simulink model "model_in_simulink"  (R2017a)
settings: Solver=FixedStepAuto  StartTime=0.0  StopTime=36*5  FixedStep=0.005  RelTol=1e-3
values from neighbouring files (symbols this model uses):
  a = theta(:,6)    [estimate_BP.m]
  alpha_Gain = theta(:,1)    [estimate_BP.m]
  alpha_Loss = theta(:,2)    [estimate_BP.m]
  b = theta(:,7)    [estimate_BP.m]
  beta_v = theta(:,9)    [estimate_BP.m]
  BP0 = theta(:,14)    [estimate_BP.m]    (also in example_crystalloid_input.mat = 97)
  BP_Target = BP0    [estimate_BP.m]
  BV0 = theta(:,11)    [estimate_BP.m]    (also in example_crystalloid_input.mat = 1.88949226726; kinetics_transition.m = req_params(4); run_main_Unified_Framework.m = temp_VSUBJECTS_VALID(i,11); run_observer.m = VSUBJECTS_NAT(i,11))
  CO0 = theta(:,13)    [estimate_BP.m]    (also in example_crystalloid_input.mat = 4.9)
  CP0 = 6    [estimate_BP.m]
  EQM = 1    [estimate_BP.m]
  Hemorrhage_inp = [0.08 0.08 0.08 0.08 0.08 0.08 0.08 0.08 0.08 0.08 0.08 0.08 ... (18001 elements, 18001x1)]    [example_crystalloid_input.mat]
  Infusion_inp = [0 0 0 0 0 0 0 0 0 0 0 0 ... (18001 elements, 18001x1)]    [example_crystalloid_input.mat]
  Ka = theta(:,4)    [estimate_BP.m]
  Kco = theta(:,10)    [estimate_BP.m]
  Kp = theta(:,3)    [estimate_BP.m]
  Ktp = theta(:,8)    [estimate_BP.m]
  Kv = theta(:,5)    [estimate_BP.m]
  R = (BP0-CP0)./CO0    [estimate_BP.m]    (also in run_EKF.m = 0.1*noise; run_UKF.m = 0.1*noise)
  Urine_inp = [0.0118 0.0118 0.0118 0.0118 0.0118 0.0118 0.0118 0.0118 0.0118 0.0118 0.0118 0.0118 ... (18001 elements, 18001x1)]    [example_crystalloid_input.mat]
undefined symbols (not defined in the file or in its folder): RB0, VA0, VV0
libraries: simulink x3
settings Model: Creator=Xin  LastModifiedBy=tivay

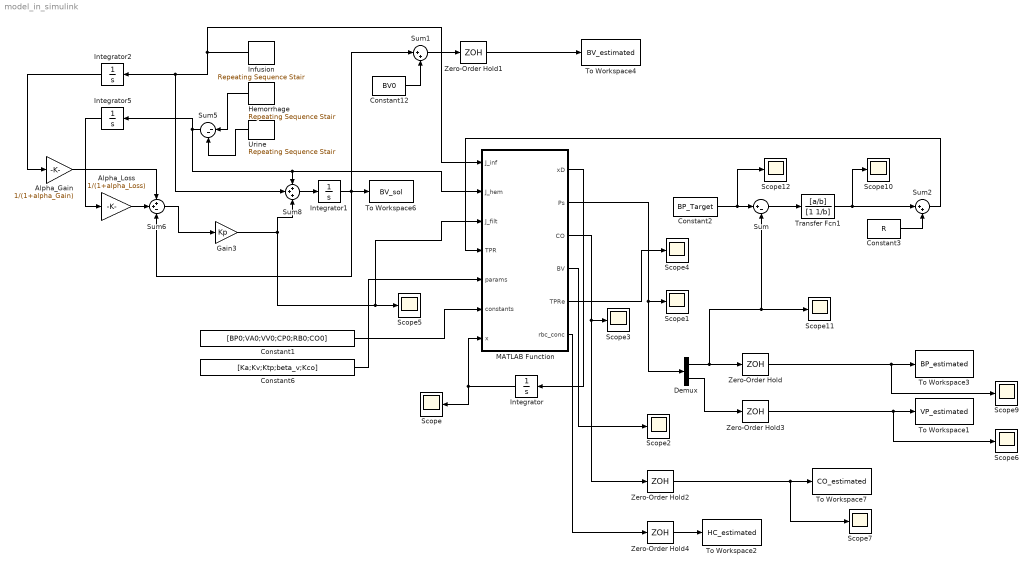
== system model_in_simulink ==
  Alpha_Gain : Gain  Gain=1/(1+alpha_Gain)
  Alpha_Loss : Gain  Gain=1/(1+alpha_Loss)
  Constant1 : Constant  Value=[BP0;VA0;VV0;CP0;RB0;CO0]  VectorParams1D=off
  Constant12 : Constant  Value=BV0
  Constant2 : Constant  Value=BP_Target
  Constant3 : Constant  Value=R
  Constant6 : Constant  Value=[Ka;Kv;Ktp;beta_v;Kco]  VectorParams1D=off
  Demux : Demux  Outputs=2
  Gain3 : Gain  Gain=Kp
  Hemorrhage : simulink/Sources/Repeating Sequence Stair  OutValues=Hemorrhage_inp*EQM  tsamp=SamplingTime  OutMin=[]  OutMax=[]  OutDataTypeStr=double  OutputDataTypeScalingMode=double  OutDataType=fixdt(0,8)  ConRadixGroup=Best Precision: Vector-wise  OutScaling=2^-12
  Infusion : simulink/Sources/Repeating Sequence Stair  OutValues=Infusion_inp*EQM  tsamp=SamplingTime  OutMin=[]  OutMax=[]  OutDataTypeStr=double  OutputDataTypeScalingMode=double  OutDataType=fixdt(0,8)  ConRadixGroup=Best Precision: Vector-wise  OutScaling=2^-12
  Integrator : Integrator  InitialCondition=[VA0;VV0;RB0;CO0]
  Integrator1 : Integrator
  Integrator2 : Integrator
  Integrator5 : Integrator
  MATLAB Function : MATLAB Function  TreatAsAtomicUnit=on
  Scope{,1..7,9..12} (12 alike) : Scope
  Sum : Sum  Inputs=|+-
  Sum1 : Sum  Inputs=|++
  Sum2 : Sum  Inputs=|++
  Sum5 : Sum  Inputs=|--
  Sum6 : Sum  Inputs=++-
  Sum8 : Sum  Inputs=+++
  To Workspace1 : ToWorkspace  VariableName=VP_estimated  SaveFormat=Timeseries  SampleTime=-1
  To Workspace2 : ToWorkspace  VariableName=HC_estimated  SaveFormat=Timeseries  SampleTime=-1
  To Workspace3 : ToWorkspace  VariableName=BP_estimated  SaveFormat=Timeseries  SampleTime=-1
  To Workspace4 : ToWorkspace  VariableName=BV_estimated  SaveFormat=Timeseries  SampleTime=-1
  To Workspace6 : ToWorkspace  VariableName=BV_sol  SampleTime=-1
  To Workspace7 : ToWorkspace  VariableName=CO_estimated  SaveFormat=Timeseries  SampleTime=-1
  Transfer Fcn1 : TransferFcn  Numerator=[a/b]  Denominator=[1 1/b]
  Urine : simulink/Sources/Repeating Sequence Stair  OutValues=Urine_inp*EQM  tsamp=SamplingTime  OutMin=[]  OutMax=[]  OutDataTypeStr=double  OutputDataTypeScalingMode=double  OutDataType=fixdt(0,8)  ConRadixGroup=Best Precision: Vector-wise  OutScaling=2^-12
  Zero-Order Hold{,1..4} (5 alike) : ZeroOrderHold  SampleTime=5
  wires:
  Sum1/1 -> Zero-Order Hold1/1
  Integrator1/1 -> Sum6/3, Sum1/1, To Workspace6/1
  Sum6/1 -> Gain3/1
  Sum8/1 -> Integrator1/1
  Integrator2/1 -> Alpha_Gain/1
  Alpha_Gain/1 -> Sum6/1
  Integrator5/1 -> Alpha_Loss/1
  Alpha_Loss/1 -> Sum6/2
  Hemorrhage/1 -> Sum5/1
  Urine/1 -> Sum5/2
  Gain3/1 -> Sum8/3, Scope5/1, MATLAB Function/3(J_filt)
  Constant12/1 -> Sum1/2
  Zero-Order Hold1/1 -> To Workspace4/1
  MATLAB Function/3(CO) -> Zero-Order Hold2/1, Scope3/1
  MATLAB Function/2(Ps) -> Demux/1, Scope1/1
  MATLAB Function/1(xD) -> Integrator/1
  Integrator/1 -> Scope/1, MATLAB Function/7(x)
  MATLAB Function/4(BV) -> Scope2/1
  Constant6/1 -> MATLAB Function/5(params)
  Demux/1 -> Sum/2, Scope11/1, Zero-Order Hold/1
  Demux/2 -> Zero-Order Hold3/1
  Constant1/1 -> MATLAB Function/6(constants)
  Transfer Fcn1/1 -> Sum2/1, Scope10/1
  Constant2/1 -> Scope12/1, Sum/1
  Sum/1 -> Transfer Fcn1/1
  Constant3/1 -> Sum2/2
  MATLAB Function/5(TPRe) -> Scope4/1
  Sum2/1 -> MATLAB Function/4(TPR)
  Sum5/1 -> Integrator5/1, MATLAB Function/2(J_hem), Sum8/1
  Infusion/1 -> MATLAB Function/1(J_inf), Integrator2/1, Sum8/2
  Zero-Order Hold/1 -> Scope9/1, To Workspace3/1
  Zero-Order Hold3/1 -> Scope6/1, To Workspace1/1
  Zero-Order Hold2/1 -> To Workspace7/1, Scope7/1
  Zero-Order Hold4/1 -> To Workspace2/1
  MATLAB Function/6(rbc_conc) -> Zero-Order Hold4/1

== matlab function model_in_simulink/MATLAB Function ==
  data: J_inf input; J_hem input; J_filt input; TPR input; params input; constants input; x input; xD output; Ps output; CO output; BV output; TPRe output; rbc_conc output
function [ xD, Ps, CO, BV, TPRe, rbc_conc ] = fcn(J_inf, J_hem, J_filt, TPR, params, constants, x)

    Va = x(1); % l
    Vv = x(2); % l
    Vr = x(3); % l
    CO = x(4); % l/m
    
    % Constants
    BP0 = constants(1);
    VA0 = constants(2);
    VV0 = constants(3);
    CP0 = constants(4);
    RB0 = constants(5);
    CO0 = constants(6);
    
    % Params
    Ka = params(1);
    Kv = params(2);
    Ktp = params(3);
    Kaa = Ka*Kv;
    
    beta_v = params(4);
    Kco = params(5);

    % Pressures
    Pa = Kaa * (Va - VA0) + BP0;
    Pv = Kv * (Vv - VV0) + CP0;
    
    % TPR
    rbc_conc_0 = RB0/(VA0+VV0);
    rbc_conc   = Vr/(Va+Vv);
    TPRe = TPR + Ktp * (rbc_conc - rbc_conc_0);
    
    % CO
    dist = beta_v * (Pv - CP0);
    coD = Kco * ( CO0 - CO - dist );
    CO = CO + dist;
    
    % Fluid Balance
    xD1 = CO - (Pa-Pv)/TPRe + J_hem + J_filt;
    xD2 = - CO + (Pa-Pv)/TPRe + J_inf;
    xD3 = + J_hem * (Vr/(Vv+Va));
    
    xD = [xD1; xD2; xD3; coD];
    Ps = [Pa; Pv];
    BV = Va + Vv;
    
end
